simulink model "lqr_sim"  (R2018b)
settings: Solver=ode4  StartTime=0.0  StopTime=sim_time  FixedStep=Ts  RelTol=1e-3
values from neighbouring files (symbols this model uses):
  A = [-0.5423,             0,             0,             0,             0,               0,             0,             0,             0,             0,        0.3395,             0 ... (first row only)    [lqr_design.m]
  B = rho*V*g*1.4    (= 168.9282)    [launcher_ROV_sim.m]    (also in lqr_design.m = [0.05581,         0,         0,         0,         0,       )
  C = [zeros(6) eye(6)]    [lqr_design.m]
  D = zeros(6,6)    [lqr_design.m]
  Kq = [-14.0522937866 -0.000724361189881 7.36173354264e-14 -0.00802187271501 -1.59153029576 -0.00240388685004 -0.00102573418256 -14.0209983601 3.7395785387e-14 1.84702452338 0.00611607698573 0.00818162190067 ... (36 elements, 6x6)]    [lqr.mat]    (also in lqr_design.m = K(:,13:end))
  Kx = [30.0077125539 0.00159520383282 -9.18372190817e-14 0.0101724452135 3.59932945814 0.00293162043647 0.00170650423442 25.0803818094 -2.91671924306e-14 -3.06896094423 -0.00658141948351 -0.00836683203268 ... (72 elements, 6x12)]    [lqr.mat]    (also in lqr_design.m = K(:,1:12))
  Ts = 0.01    [launcher_ROV_sim.m]    (also in lqr_design.m)
  x0 = [0, 0, 0, 0, 0, 0, 0, 0, 0, 0, 0, 0]'    [lqr_design.m]
libraries: aerolibanim x2, cstblocks x1
settings Model: Creator=d066103  LastModifiedBy=corra
settings DebuggingCC: SFMachineParentedDataDiag=error

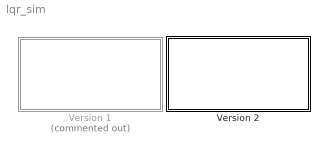
== system lqr_sim ==
  Version 1 : Subsystem  Commented=on
  Version 2 : Subsystem

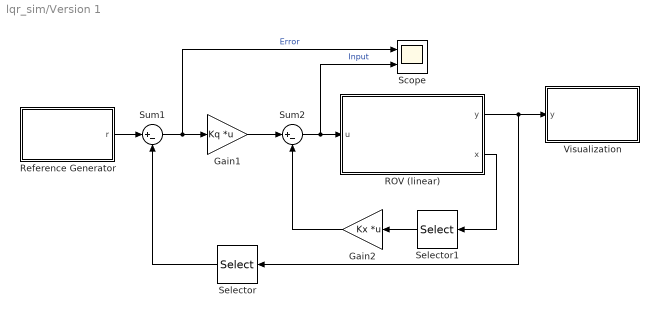
== system lqr_sim/Version 1 ==
  Gain1 : Gain  Gain=Kq  Multiplication=Matrix(K*u)
  Gain2 : Gain  Gain=Kx  Multiplication=Matrix(K*u)
  ROV (linear) : Subsystem
  Reference Generator : Subsystem
  Scope : Scope  NumInputPorts=2
  Selector : Selector  InputPortWidth=12  IndexOptions=Index vector (dialog)  Indices=[7:12]  OutputSizes=1
  Selector1 : Selector  InputPortWidth=12  IndexOptions=Index vector (dialog)  Indices=[1:6]  OutputSizes=1
  Sum1 : Sum  Inputs=|+-
  Sum2 : Sum  Inputs=|+-
  Visualization : Subsystem
  wires:
  Gain2/1 -> Sum2/2
  Reference Generator/1(r) -> Sum1/1
  Sum2/1 -> ROV (linear)/1(u), Scope/2  "Input"
  Gain1/1 -> Sum2/1
  Sum1/1 -> Gain1/1, Scope/1  "Error"
  ROV (linear)/1(y) -> Selector/1, Visualization/1(y)
  ROV (linear)/2(x) -> Selector1/1
  Selector/1 -> Sum1/2
  Selector1/1 -> Gain2/1

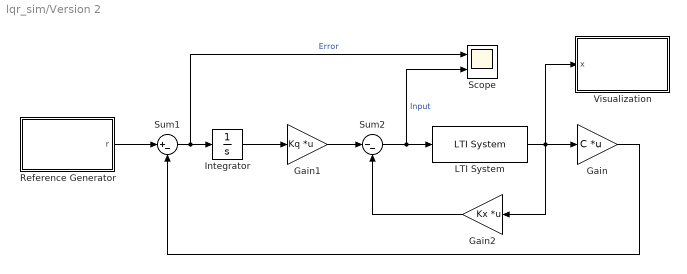
== system lqr_sim/Version 2 ==
  Gain : Gain  Gain=C  Multiplication=Matrix(K*u)
  Gain1 : Gain  Gain=Kq  Multiplication=Matrix(K*u)
  Gain2 : Gain  Gain=Kx  Multiplication=Matrix(K*u)
  Integrator : Integrator
  LTI System : cstblocks/LTI System  sys=sys_x  IC=[]
  Reference Generator : Subsystem
  Scope : Scope  NumInputPorts=2
  Sum1 : Sum  Inputs=|+-
  Sum2 : Sum  Inputs=|--
  Visualization : Subsystem
  wires:
  Gain/1 -> Sum1/2
  Reference Generator/1(r) -> Sum1/1
  LTI System/1 -> Gain2/1, Gain/1, Visualization/1(x)
  Gain1/1 -> Sum2/1
  Sum2/1 -> LTI System/1, Scope/2  "Input"
  Gain2/1 -> Sum2/2
  Integrator/1 -> Gain1/1
  Sum1/1 -> Scope/1, Integrator/1  "Error"

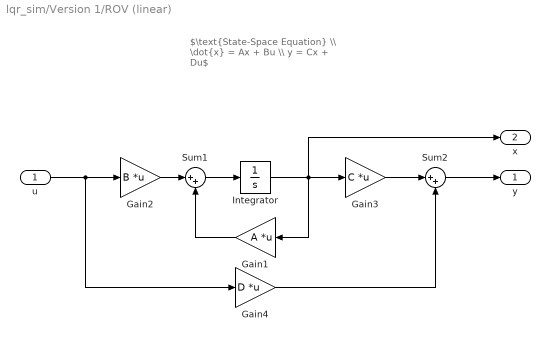
== system lqr_sim/Version 1/ROV (linear) ==
  note: $\text{State-Space Equation} \\ \dot{x} = Ax + Bu \\ y = Cx + Du$
  u : Inport  PortDimensions=6
  Gain1 : Gain  Gain=A  Multiplication=Matrix(K*u)
  Gain2 : Gain  Gain=B  Multiplication=Matrix(K*u)
  Gain3 : Gain  Gain=C  Multiplication=Matrix(K*u)
  Gain4 : Gain  Gain=D  Multiplication=Matrix(K*u)
  Integrator : Integrator  InitialCondition=x0
  Sum1 : Sum  Inputs=|++
  Sum2 : Sum  Inputs=|++
  y : Outport  PortDimensions=12
  x : Outport  Port=2  PortDimensions=12
  wires:
  Gain2/1 -> Sum1/1
  Sum2/1 -> y/1
  Gain4/1 -> Sum2/2
  u/1 -> Gain2/1, Gain4/1
  Gain3/1 -> Sum2/1
  Sum1/1 -> Integrator/1
  Integrator/1 -> x/1, Gain1/1, Gain3/1
  Gain1/1 -> Sum1/2

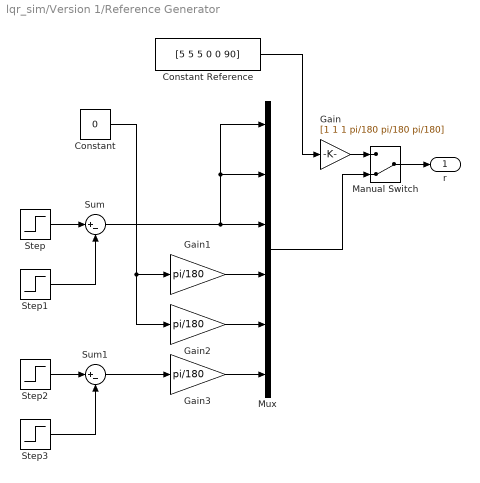
== system lqr_sim/Version 1/Reference Generator ==
  Constant : Constant  Value=0
  Constant Reference : Constant  Value=[5 5 5 0 0 90]
  Gain : Gain  Gain=[1 1 1 pi/180 pi/180 pi/180]
  Gain1 : Gain  Gain=pi/180
  Gain2 : Gain  Gain=pi/180
  Gain3 : Gain  Gain=pi/180
  Manual Switch : ManualSwitch  CurrentSetting=0
  Mux : Mux  Inputs=6
  Step : Step  Time=10  After=5  SampleTime=0
  Step1 : Step  Time=60  After=5  SampleTime=0
  Step2 : Step  Time=10  After=90  SampleTime=0
  Step3 : Step  Time=60  After=90  SampleTime=0
  Sum : Sum  Inputs=|+-
  Sum1 : Sum  Inputs=|+-
  r : Outport
  wires:
  Constant Reference/1 -> Gain/1
  Manual Switch/1 -> r/1
  Mux/1 -> Manual Switch/2
  Sum/1 -> Mux/1, Mux/2, Mux/3
  Constant/1 -> Gain1/1, Gain2/1
  Step/1 -> Sum/1
  Step1/1 -> Sum/2
  Gain/1 -> Manual Switch/1
  Gain1/1 -> Mux/4
  Gain2/1 -> Mux/5
  Gain3/1 -> Mux/6
  Step3/1 -> Sum1/2
  Step2/1 -> Sum1/1
  Sum1/1 -> Gain3/1

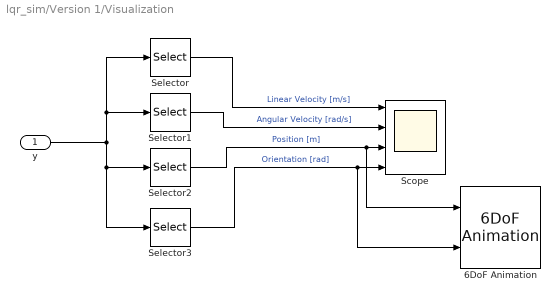
== system lqr_sim/Version 1/Visualization ==
  y : Inport
  6DoF Animation : aerolibanim/6DoF Animation  u1=[-25 25 -25 25 -25 25]  u2=10*Ts  u3=20  u4=[5000 5000 5000]  u5=Fixed position  u6=[200 250 -200]  u7=10  u8=on
      settings: SourceProductName=Aerospace Blockset
  Scope : Scope  NumInputPorts=4
  Selector : Selector  InputPortWidth=12  IndexOptions=Index vector (dialog)  Indices=[1:3]  OutputSizes=1
  Selector1 : Selector  InputPortWidth=12  IndexOptions=Index vector (dialog)  Indices=[4:6]  OutputSizes=1
  Selector2 : Selector  InputPortWidth=12  IndexOptions=Index vector (dialog)  Indices=[7:9]  OutputSizes=1
  Selector3 : Selector  InputPortWidth=12  IndexOptions=Index vector (dialog)  Indices=[10:12]  OutputSizes=1
  wires:
  Selector1/1 -> Scope/2  "Angular Velocity [rad/s]"
  Selector3/1 -> 6DoF Animation/2, Scope/4  "Orientation [rad]"
  Selector/1 -> Scope/1  "Linear Velocity [m/s]"
  Selector2/1 -> 6DoF Animation/1, Scope/3  "Position [m]"
  y/1 -> Selector/1, Selector1/1, Selector3/1, Selector2/1

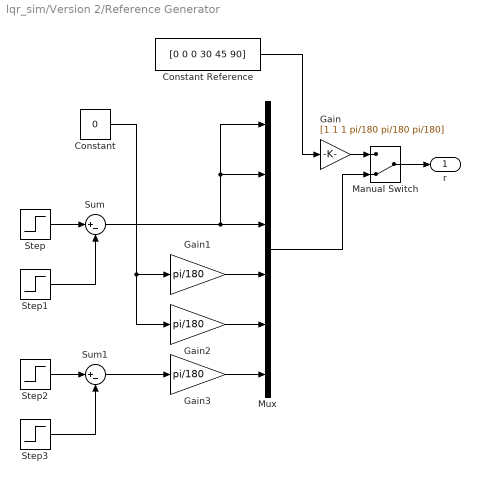
== system lqr_sim/Version 2/Reference Generator ==
  Constant : Constant  Value=0
  Constant Reference : Constant  Value=[0 0 0 30 45 90]
  Gain : Gain  Gain=[1 1 1 pi/180 pi/180 pi/180]
  Gain1 : Gain  Gain=pi/180
  Gain2 : Gain  Gain=pi/180
  Gain3 : Gain  Gain=pi/180
  Manual Switch : ManualSwitch  CurrentSetting=0
  Mux : Mux  Inputs=6
  Step : Step  Time=10  After=5  SampleTime=0
  Step1 : Step  Time=60  After=5  SampleTime=0
  Step2 : Step  Time=10  After=90  SampleTime=0
  Step3 : Step  Time=60  After=90  SampleTime=0
  Sum : Sum  Inputs=|+-
  Sum1 : Sum  Inputs=|+-
  r : Outport
  wires:
  Constant Reference/1 -> Gain/1
  Manual Switch/1 -> r/1
  Mux/1 -> Manual Switch/2
  Sum/1 -> Mux/1, Mux/2, Mux/3
  Constant/1 -> Gain1/1, Gain2/1
  Step/1 -> Sum/1
  Step1/1 -> Sum/2
  Gain/1 -> Manual Switch/1
  Gain1/1 -> Mux/4
  Gain2/1 -> Mux/5
  Gain3/1 -> Mux/6
  Step3/1 -> Sum1/2
  Step2/1 -> Sum1/1
  Sum1/1 -> Gain3/1

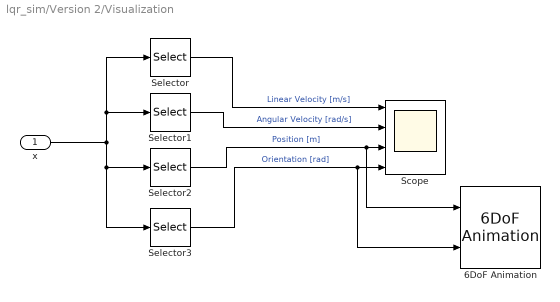
== system lqr_sim/Version 2/Visualization ==
  x : Inport
  6DoF Animation : aerolibanim/6DoF Animation  u1=[-25 25 -25 25 -25 25]  u2=10*Ts  u3=20  u4=[5000 5000 5000]  u5=Fixed position  u6=[200 250 -200]  u7=10  u8=on
      settings: SourceProductName=Aerospace Blockset
  Scope : Scope  NumInputPorts=4
  Selector : Selector  InputPortWidth=12  IndexOptions=Index vector (dialog)  Indices=[1:3]  OutputSizes=1
  Selector1 : Selector  InputPortWidth=12  IndexOptions=Index vector (dialog)  Indices=[4:6]  OutputSizes=1
  Selector2 : Selector  InputPortWidth=12  IndexOptions=Index vector (dialog)  Indices=[7:9]  OutputSizes=1
  Selector3 : Selector  InputPortWidth=12  IndexOptions=Index vector (dialog)  Indices=[10:12]  OutputSizes=1
  wires:
  Selector1/1 -> Scope/2  "Angular Velocity [rad/s]"
  Selector3/1 -> 6DoF Animation/2, Scope/4  "Orientation [rad]"
  Selector/1 -> Scope/1  "Linear Velocity [m/s]"
  Selector2/1 -> 6DoF Animation/1, Scope/3  "Position [m]"
  x/1 -> Selector/1, Selector1/1, Selector3/1, Selector2/1
